simulink model "chuanbing"  (R2016b)
settings: Solver=VariableStepAuto  StartTime=0.0  StopTime=1  RelTol=1e-3
libraries: commrandsrc3 x3, commsrccod2 x1, dsparch4 x1, commutil2 x1
settings Model: Creator=white  LastModifiedBy=white

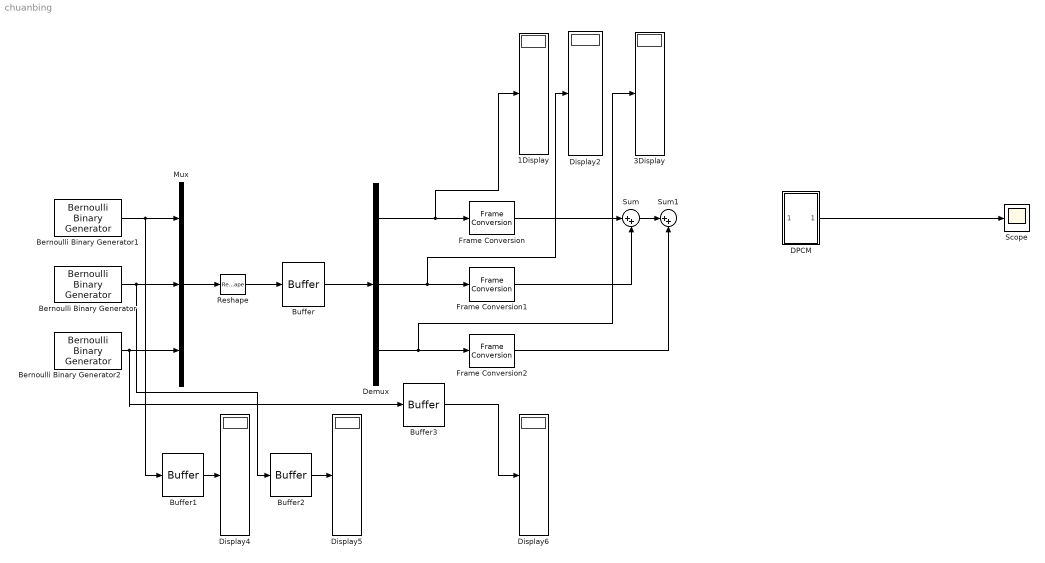
== system chuanbing ==
  1Display : Display
      settings: Format=binary (Stored Integer)
  3Display : Display
      settings: Format=binary (Stored Integer)
  Bernoulli Binary Generator : commrandsrc3/Bernoulli Binary Generator  ProbabilityOfZero=0.5  SeedSource=Auto  Seed=0  SampleTime=1/8  SamplesPerFrame=1  OutputDataType=double  SimulateUsing=Interpreted execution
  Bernoulli Binary Generator1 : commrandsrc3/Bernoulli Binary Generator  ProbabilityOfZero=0.5  SeedSource=Auto  Seed=0  SampleTime=1/8  SamplesPerFrame=1  OutputDataType=double  SimulateUsing=Interpreted execution
  Bernoulli Binary Generator2 : commrandsrc3/Bernoulli Binary Generator  ProbabilityOfZero=0.5  SeedSource=Auto  Seed=0  SampleTime=1/8  SamplesPerFrame=1  OutputDataType=double  SimulateUsing=Interpreted execution
  Buffer : Buffer  N=24  TreatMby1Signals=One channel  OutputFrames=off
  Buffer1 : Buffer  N=8  TreatMby1Signals=One channel  OutputFrames=off
  Buffer2 : Buffer  N=8  TreatMby1Signals=One channel  OutputFrames=off
  Buffer3 : Buffer  N=8  TreatMby1Signals=One channel  OutputFrames=off
  "DPCM " : Subsystem
  Demux : Demux  Outputs=3
  Display{2,4..6} (4 alike) : Display
      settings: Format=binary (Stored Integer)
  Frame Conversion : FrameConversion  InheritSamplingMode=off
  Frame Conversion1 : FrameConversion  InheritSamplingMode=off
  Frame Conversion2 : FrameConversion  InheritSamplingMode=off
  Mux : Mux  Inputs=3
  Reshape : Reshape
  Scope : Scope
  Sum : Sum  Inputs=|++
  Sum1 : Sum  Inputs=|++
  wires:
  Buffer/1 -> Demux/1
  Demux/2 -> Frame Conversion1/1, Display2/1
  Demux/3 -> 3Display/1, Frame Conversion2/1
  Demux/1 -> Frame Conversion/1, 1Display/1
  Frame Conversion/1 -> Sum/1
  Frame Conversion1/1 -> Sum/2
  Sum/1 -> Sum1/1
  Frame Conversion2/1 -> Sum1/2
  "DPCM "/1(Out1) -> Scope/1
  Bernoulli Binary Generator1/1 -> Buffer1/1, Mux/1
  Bernoulli Binary Generator/1 -> Buffer2/1, Mux/2
  Bernoulli Binary Generator2/1 -> Buffer3/1, Mux/3
  Mux/1 -> Reshape/1
  Reshape/1 -> Buffer/1
  Buffer1/1 -> Display4/1
  Buffer2/1 -> Display5/1
  Buffer3/1 -> Display6/1

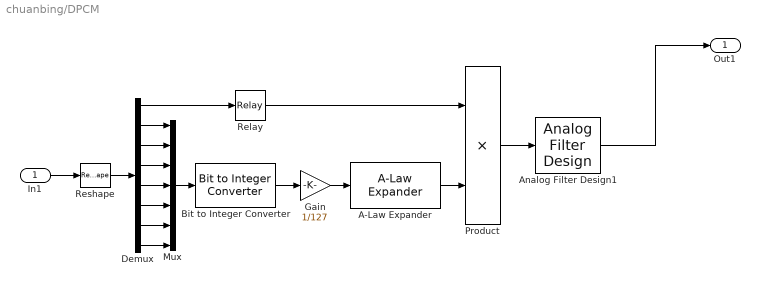
== system chuanbing/DPCM  ==
  In1 : Inport
  A-Law Expander : commsrccod2/A-Law Expander  A=87.6  V=1
  Analog Filter Design1 : dsparch4/Analog Filter Design  method=Butterworth  filttype=Lowpass  N=8  Wlo=2*120*pi  Whi=80  Rp=2  Rs=40
  Bit to Integer Converter : commutil2/Bit to Integer Converter  nbits=7  bitOrder=MSB first  signedOutputValues=Unsigned  outDtype=Inherit via internal rule  outDtypeSigned=Inherit via internal rule
  Demux : Demux  Outputs=8
  Gain : Gain  Gain=1/127
  Mux : Mux  Inputs=7
  Product : Product
  Relay : Relay  OnSwitchValue=0.5  OffSwitchValue=0.5  OnOutputValue=-1  OffOutputValue=1
  Reshape : Reshape
  Out1 : Outport
  wires:
  Demux/2 -> Mux/1
  Demux/3 -> Mux/2
  Demux/4 -> Mux/3
  Demux/5 -> Mux/4
  Demux/6 -> Mux/5
  Demux/7 -> Mux/6
  Demux/8 -> Mux/7
  Bit to Integer Converter/1 -> Gain/1
  Mux/1 -> Bit to Integer Converter/1
  Relay/1 -> Product/1
  Gain/1 -> A-Law Expander/1
  Demux/1 -> Relay/1
  A-Law Expander/1 -> Product/2
  Reshape/1 -> Demux/1
  Product/1 -> Analog Filter Design1/1
  In1/1 -> Reshape/1
  Analog Filter Design1/1 -> Out1/1
